simulink model "RL_Resource_Allocation"  (R2023b)
settings: Solver=FixedStepAuto  StartTime=0.0  StopTime=inf  FixedStep=Ts  RelTol=1e-3
values from neighbouring files (symbols this model uses):
  doTraining = false    [ResourceAllocation_ddpg.m]    (also in ResourceAllocation_td3.m)
  gamma = 0:0.01:1    [GeneratingPlots_Demand_Alloc_Paper.m]    (also in ResourceAllocation_ddpg.m; ResourceAllocation_td3.m; networkResetFcn.m = round(rand,2))
  initAllocation = [25 25]*scaling_factor    [ResourceAllocation_ddpg.m]    (also in ResourceAllocation_td3.m)
  LTEDemandSeries = zeros(1,numPastDataPoints+1)    [ResourceAllocation_ddpg.m]    (also in ResourceAllocation_td3.m; networkResetFcn.m = LTEDataTimeseries.NRB(dataIndex:-1:(dataIndex-numPastDataPoi; networkResetFcnSim.m = LTEDataTimeseries.NRB(dataIndex:-1:(dataIndex-numPastDataPoi)
  LTEInitialDemand = LTEDataTimeseries.NRB(10:-1:1)    [ResourceAllocation_ddpg.m]    (also in ResourceAllocation_td3.m; networkResetFcn.m; networkResetFcnSim.m)
  N_R = [20,60,100]    [ResourceAllocation_ddpg.m]    (also in ResourceAllocation_td3.m)
  NRDemandSeries = zeros(1,numPastDataPoints+1)    [ResourceAllocation_ddpg.m]    (also in ResourceAllocation_td3.m; networkResetFcn.m = NRDataTimeseries.NRB(dataIndex:-1:(dataIndex-numPastDataPoin; networkResetFcnSim.m = NRDataTimeseries.NRB(dataIndex:-1:(dataIndex-numPastDataPoin)
  NRInitialDemand = NRDataTimeseries.NRB(10:-1:1)    [ResourceAllocation_ddpg.m]    (also in ResourceAllocation_td3.m; networkResetFcn.m; networkResetFcnSim.m)
  numPastDataPoints = 10    [ResourceAllocation_ddpg.m]    (also in ResourceAllocation_td3.m)
libraries: rllib x1
settings Model: Creator=sng29  LastModifiedBy=sng29
settings DebuggingCC: AlgebraicLoopMsg=none

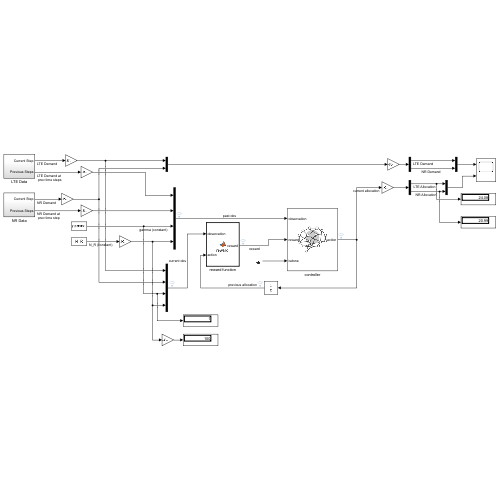
[thumbnail: Simulink's stored preview of the top-level diagram]
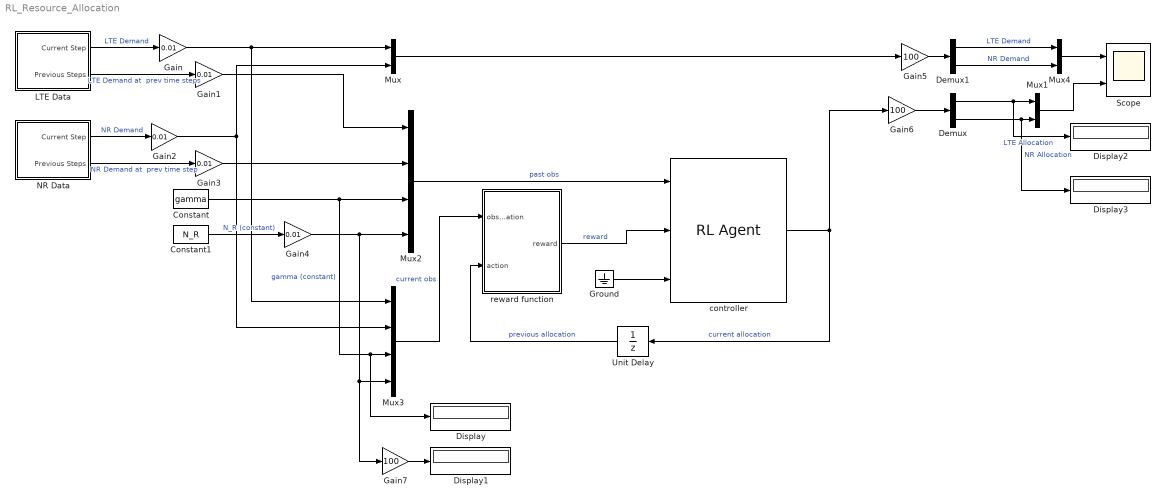
== system RL_Resource_Allocation ==
  Constant : Constant  Value=gamma
  Constant1 : Constant  Value=N_R
  Demux : Demux  Outputs=2
  Demux1 : Demux  Outputs=2
  Display{,1..3} (4 alike) : Display
  Gain{,1..4} (5 alike) : Gain  Gain=0.01
  Gain5 : Gain  Gain=100
  Gain6 : Gain  Gain=100
  Gain7 : Gain  Gain=100
  Ground : Ground
  LTE Data : Subsystem
  Mux : Mux  Inputs=2
  Mux1 : Mux  Inputs=2
  Mux2 : Mux
  Mux3 : Mux
  Mux4 : Mux  Inputs=2
  NR Data : Subsystem
  Scope : Scope  NumInputPorts=2
  Unit Delay : UnitDelay  InitialCondition=initAllocation  SampleTime=-1  HasFrameUpgradeWarning=on
  controller : rllib/RL Agent  Agent=agent  ExternalActionAsInput=off  ProvideLastAction=off  ProvideCumRwd=off  TreatAsDirectFeedthrough=on  UseStrictObservationDataTypes=off
  reward function : MATLAB Function  TreatAsAtomicUnit=on
  wires:
  reward function/1(reward) -> controller/2  "reward"
  Ground/1 -> controller/3
  Unit Delay/1 -> reward function/2(action)  "previous allocation"
  Mux3/1 -> reward function/1(observation)  "current obs"
  Mux1/1 -> Scope/2
  Demux/1 -> Mux1/1, Display2/1  "LTE Allocation"
  Demux/2 -> Mux1/2, Display3/1  "NR Allocation"
  Constant/1 -> Display/1, Mux3/3, Mux2/3  "gamma (constant)"
  Mux2/1 -> controller/1  "past obs"
  Constant1/1 -> Gain4/1  "N_R (constant)"
  LTE Data/2(Previous Steps) -> Gain1/1  "LTE Demand at  prev time steps"
  NR Data/2(Previous Steps) -> Gain3/1  "NR Demand at  prev time step"
  controller/1 -> Unit Delay/1, Gain6/1  "current allocation"
  LTE Data/1(Current Step) -> Gain/1  "LTE Demand"
  NR Data/1(Current Step) -> Gain2/1  "NR Demand"
  Mux/1 -> Gain5/1
  Gain/1 -> Mux3/1, Mux/1
  Gain1/1 -> Mux2/1
  Gain2/1 -> Mux3/2, Mux/2
  Gain3/1 -> Mux2/2
  Gain4/1 -> Gain7/1, Mux3/4, Mux2/4
  Gain5/1 -> Demux1/1
  Gain6/1 -> Demux/1
  Gain7/1 -> Display1/1
  Demux1/1 -> Mux4/1  "LTE Demand"
  Demux1/2 -> Mux4/2  "NR Demand"
  Mux4/1 -> Scope/1

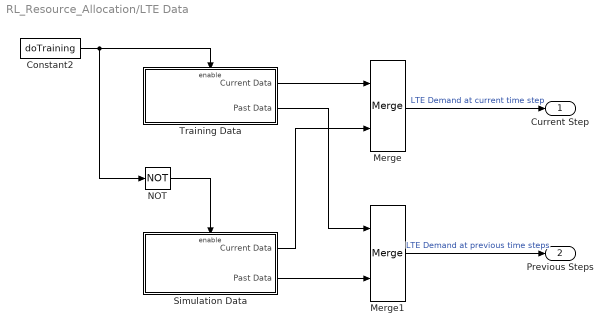
== system RL_Resource_Allocation/LTE Data ==
  Constant2 : Constant  Value=doTraining
  Merge : Merge
  Merge1 : Merge
  NOT : Logic  Operator=NOT  AllPortsSameDT=off  OutDataTypeStr=boolean
  Simulation Data : Subsystem  TreatAsAtomicUnit=on
  Training Data : Subsystem  TreatAsAtomicUnit=on
  Current Step : Outport
  Previous Steps : Outport  Port=2
  wires:
  Constant2/1 -> Training Data/Enable, NOT/1
  Merge/1 -> Current Step/1  "LTE Demand at current time step"
  Merge1/1 -> Previous Steps/1  "LTE Demand at previous time steps"
  Training Data/1(Current Data) -> Merge/1
  Training Data/2(Past Data) -> Merge1/1
  NOT/1 -> Simulation Data/Enable
  Simulation Data/1(Current Data) -> Merge/2
  Simulation Data/2(Past Data) -> Merge1/2

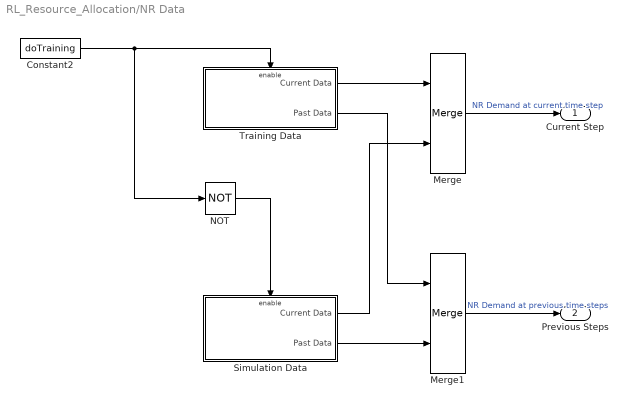
== system RL_Resource_Allocation/NR Data ==
  Constant2 : Constant  Value=doTraining
  Merge : Merge
  Merge1 : Merge
  NOT : Logic  Operator=NOT  AllPortsSameDT=off  OutDataTypeStr=boolean
  Simulation Data : Subsystem  TreatAsAtomicUnit=on
  Training Data : Subsystem  TreatAsAtomicUnit=on
  Current Step : Outport
  Previous Steps : Outport  Port=2
  wires:
  Constant2/1 -> Training Data/Enable, NOT/1
  Merge/1 -> Current Step/1  "NR Demand at current time step"
  Merge1/1 -> Previous Steps/1  "NR Demand at previous time steps"
  Training Data/1(Current Data) -> Merge/1
  NOT/1 -> Simulation Data/Enable
  Simulation Data/1(Current Data) -> Merge/2
  Simulation Data/2(Past Data) -> Merge1/2
  Training Data/2(Past Data) -> Merge1/1

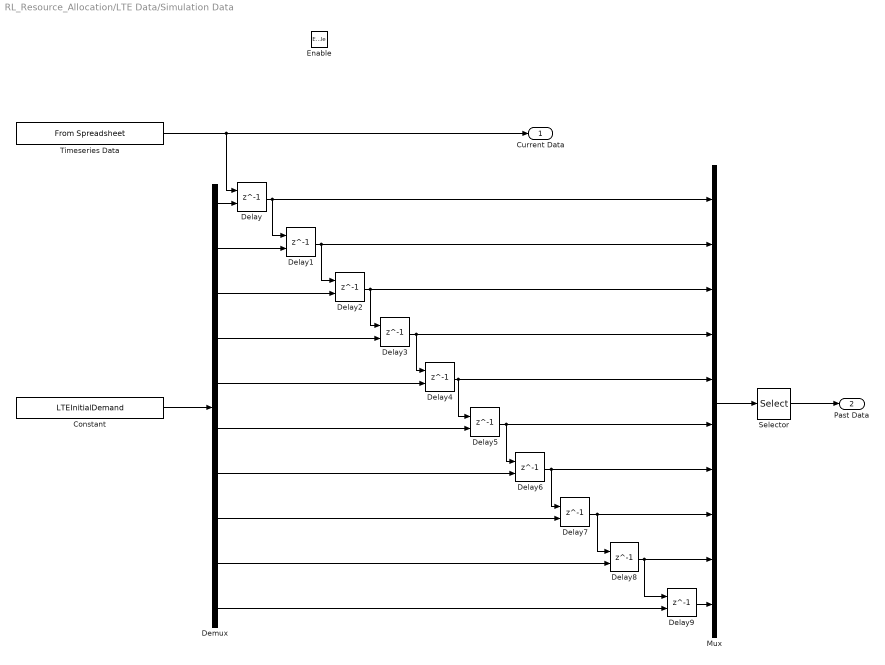
== system RL_Resource_Allocation/LTE Data/Simulation Data ==
  Enable : EnablePort
  Constant : Constant  Value=LTEInitialDemand
  Delay{,1..9} (10 alike) : Delay  DelayLength=1  InitialConditionSource=Input port
      settings: InputPortMap=u0,p4
  Demux : Demux  Outputs=10
  Mux : Mux  Inputs=10
  Selector : Selector  InputPortWidth=10  IndexOptions=Index vector (dialog)  Indices=1:numPastDataPoints  OutputSizes=1
  Timeseries Data : FromSpreadsheet  FileName=LTE_Demand_0.xlsx  SheetName=Output_2115_hourly  Range=B1:B861  TreatFirstColumnAs=Data  SampleTime=1  OutputAfterLastPoint=Hold final value
  Current Data : Outport
  Past Data : Outport  Port=2
  wires:
  Delay9/1 -> Mux/10
  Delay4/1 -> Delay5/1, Mux/5
  Delay2/1 -> Delay3/1, Mux/3
  Constant/1 -> Demux/1
  Delay8/1 -> Delay9/1, Mux/9
  Delay7/1 -> Delay8/1, Mux/8
  Delay/1 -> Delay1/1, Mux/1
  Timeseries Data/1 -> Current Data/1, Delay/1
  Delay6/1 -> Delay7/1, Mux/7
  Delay5/1 -> Delay6/1, Mux/6
  Delay3/1 -> Delay4/1, Mux/4
  Mux/1 -> Selector/1
  Demux/1 -> Delay/2
  Selector/1 -> Past Data/1
  Delay1/1 -> Delay2/1, Mux/2
  Demux/2 -> Delay1/2
  Demux/3 -> Delay2/2
  Demux/4 -> Delay3/2
  Demux/5 -> Delay4/2
  Demux/6 -> Delay5/2
  Demux/7 -> Delay6/2
  Demux/8 -> Delay7/2
  Demux/9 -> Delay8/2
  Demux/10 -> Delay9/2

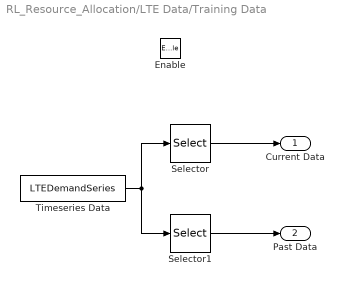
== system RL_Resource_Allocation/LTE Data/Training Data ==
  Enable : EnablePort
  Selector : Selector  InputPortWidth=numPastDataPoints + 1  IndexOptions=Index vector (dialog)  Indices=1  OutputSizes=1
  Selector1 : Selector  InputPortWidth=numPastDataPoints + 1  IndexOptions=Index vector (dialog)  Indices=2:numPastDataPoints+1  OutputSizes=1
  Timeseries Data : Constant  Value=LTEDemandSeries
  Current Data : Outport
  Past Data : Outport  Port=2
  wires:
  Selector1/1 -> Past Data/1
  Selector/1 -> Current Data/1
  Timeseries Data/1 -> Selector/1, Selector1/1

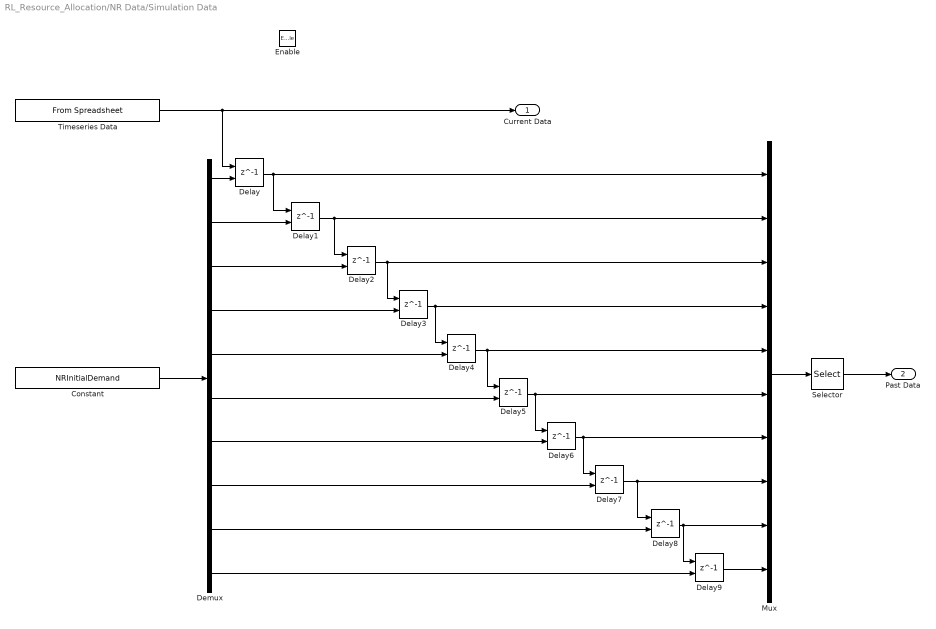
== system RL_Resource_Allocation/NR Data/Simulation Data ==
  Enable : EnablePort
  Constant : Constant  Value=NRInitialDemand
  Delay{,1..9} (10 alike) : Delay  DelayLength=1  InitialConditionSource=Input port
      settings: InputPortMap=u0,p4
  Demux : Demux  Outputs=10
  Mux : Mux  Inputs=10
  Selector : Selector  InputPortWidth=10  IndexOptions=Index vector (dialog)  Indices=1:numPastDataPoints  OutputSizes=1
  Timeseries Data : FromSpreadsheet  FileName=NR_Demand_0.xlsx  SheetName=Output_2115_hourly_NR  Range=B11:B861  TreatFirstColumnAs=Data  SampleTime=1  OutputAfterLastPoint=Hold final value
  Current Data : Outport
  Past Data : Outport  Port=2
  wires:
  Demux/1 -> Delay/2
  Constant/1 -> Demux/1
  Delay8/1 -> Mux/9, Delay9/1
  Delay9/1 -> Mux/10
  Mux/1 -> Selector/1
  Delay3/1 -> Delay4/1, Mux/4
  Delay7/1 -> Mux/8, Delay8/1
  Delay2/1 -> Mux/3, Delay3/1
  Delay5/1 -> Mux/6, Delay6/1
  Selector/1 -> Past Data/1
  Delay6/1 -> Mux/7, Delay7/1
  Delay4/1 -> Mux/5, Delay5/1
  Delay/1 -> Delay1/1, Mux/1
  Delay1/1 -> Mux/2, Delay2/1
  Timeseries Data/1 -> Current Data/1, Delay/1
  Demux/2 -> Delay1/2
  Demux/3 -> Delay2/2
  Demux/4 -> Delay3/2
  Demux/5 -> Delay4/2
  Demux/6 -> Delay5/2
  Demux/7 -> Delay6/2
  Demux/8 -> Delay7/2
  Demux/9 -> Delay8/2
  Demux/10 -> Delay9/2

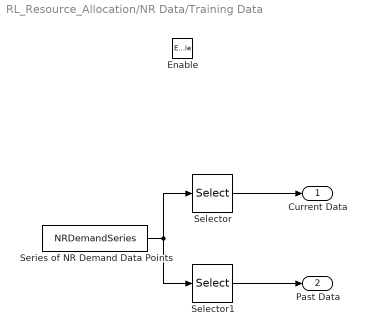
== system RL_Resource_Allocation/NR Data/Training Data ==
  Enable : EnablePort
  Selector : Selector  InputPortWidth=numPastDataPoints + 1  IndexOptions=Index vector (dialog)  Indices=1  OutputSizes=1
  Selector1 : Selector  InputPortWidth=numPastDataPoints + 1  IndexOptions=Index vector (dialog)  Indices=2:numPastDataPoints+1  OutputSizes=1
  Series of NR Demand Data Points : Constant  Value=NRDemandSeries
  Current Data : Outport
  Past Data : Outport  Port=2
  wires:
  Selector/1 -> Current Data/1
  Series of NR Demand Data Points/1 -> Selector/1, Selector1/1
  Selector1/1 -> Past Data/1

== matlab function RL_Resource_Allocation/reward function ==
  data: observation input; action input; reward output
function reward = reward(observation,action)

D_A = observation(1);
D_B = observation(2);
w_A = observation(3);
w_B = 1-w_A;
N_R = observation(4);
N_A = action(1);
N_B = action(2);

if D_A + D_B - N_R > 0
    if N_A + N_B - N_R > 0
       reward = -(w_A*(((N_A - D_A)/D_A)^2) + w_B*(((N_B - D_B)/D_B)^2)) - (10*(w_A*(((N_A - D_A)/D_A)^2) + w_B*(((N_B - D_B)/D_B)^2)));
    elseif N_A == 0 || N_B == 0 
       reward = 0;
       if N_A == 0 
          reward = reward-(w_A*(((N_A - D_A)/D_A)^2) + w_B*(((N_B - D_B)/D_B)^2)) - (5*(w_A*(((N_A - D_A)/D_A)^2) + w_B*(((N_B - D_B)/D_B)^2)));
       end
       if N_B == 0
          reward = reward-(w_A*(((N_A - D_A)/D_A)^2) + w_B*(((N_B - D_B)/D_B)^2)) - (5*(w_A*(((N_A - D_A)/D_A)^2) + w_B*(((N_B - D_B)/D_B)^2)));
       end
    elseif (N_A + N_B > N_R - 0.03 && N_A + N_B - N_R < 0)
        reward = -(w_A*(((N_A - D_A)/D_A)^2) + w_B*(((N_B - D_B)/D_B)^2)) + 10;
    else
        reward = -(w_A*(((N_A - D_A)/D_A)^2) + w_B*(((N_B - D_B)/D_B)^2)) + 5;
    end
else
    if N_A + N_B - N_R > 0
        reward = -(w_A*(((N_A - D_A)/D_A)^2) + w_B*(((N_B - D_B)/D_B)^2)) - (10*(w_A*(((N_A - D_A)/D_A)^2) + w_B*(((N_B - D_B)/D_B)^2)));
    elseif N_A - D_A < 0 || N_B - D_B < 0 || N_A - D_A > 0 || N_B - D_B > 0 || N_A == 0 || N_B == 0
        reward = 0;
        if N_A - D_A < 0
            reward = reward - (w_A*(((N_A - D_A)/D_A)^2) + w_B*(((N_B - D_B)/D_B)^2)) - (5*(w_A*(((N_A - D_A)/D_A)^2) + w_B*(((N_B - D_B)/D_B)^2)));
        end
        if N_B - D_B < 0
            reward = reward - (w_A*(((N_A - D_A)/D_A)^2) + w_B*(((N_B - D_B)/D_B)^2)) - (5*(w_A*(((N_A - D_A)/D_A)^2) + w_B*(((N_B - D_B)/D_B)^2)));
        end
        if N_A - D_A > 0
            reward = reward - (w_A*(((N_A - D_A)/D_A)^2) + w_B*(((N_B - D_B)/D_B)^2)) - (5*(w_A*(((N_A - D_A)/D_A)^2) + w_B*(((N_B - D_B)/D_B)^2)));
        end
        if N_B - D_B > 0
            reward = reward - (w_A*(((N_A - D_A)/D_A)^2) + w_B*(((N_B - D_B)/D_B)^2)) - (5*(w_A*(((N_A - D_A)/D_A)^2) + w_B*(((N_B - D_B)/D_B)^2)));
        end
        if N_A == 0
           reward = reward - (w_A*(((N_A - D_A)/D_A)^2) + w_B*(((N_B - D_B)/D_B)^2)) - (5*(w_A*(((N_A - D_A)/D_A)^2) + w_B*(((N_B - D_B)/D_B)^2)));
        end
        if N_B == 0
           reward = reward - (w_A*(((N_A - D_A)/D_A)^2) + w_B*(((N_B - D_B)/D_B)^2)) - (5*(w_A*(((N_A - D_A)/D_A)^2) + w_B*(((N_B - D_B)/D_B)^2)));
        end
    else
        reward = -(w_A*(((N_A - D_A)/D_A)^2) + w_B*(((N_B - D_B)/D_B)^2));
    end
end
